simulink model "serial_communication_simulink_model"  (Simulink 7.9)
settings: Solver=ode45  StartTime=0.0  StopTime=10.0  RelTol=1e-3
undefined symbols (not defined in the file or in its folder): LF, serial
libraries: instrumentlib x2
settings Model: Creator=Alexandre  LastModifiedBy=Alexandre

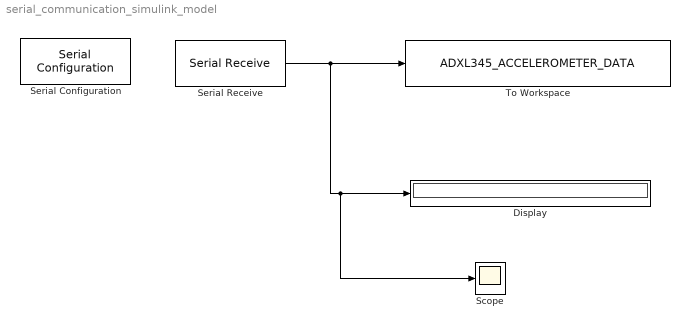
== system serial_communication_simulink_model ==
  Display : Display
  Scope : Scope
      settings: YMin=12.5  YMax=57.5
  Serial Configuration : instrumentlib/Serial Configuration  Priority=-200000  ComPortMenu=COM3  ComPort=COM3  ObjConstructor=serial('COM3');  BaudRate=9600  DataBits=8  Parity=none  StopBits=1  FlowControl=none  Timeout=10  ByteOrder=LittleEndian
  Serial Receive : instrumentlib/Serial Receive  ComPortMenu=COM3  ComPort=COM3  ObjConstructor=serial('COM3');  Terminator=LF ('\n')  DataSize="[1  3]"  DataType=uint8  EnableBlockingMode=on  ActionDataUnavailable=Output last received value  CustomValue=0  SampleTime=0.01
  To Workspace : ToWorkspace  VariableName=ADXL345_ACCELEROMETER_DATA  SampleTime=-1  SaveFormat=Structure With Time
  wires:
  Serial Receive/1 -> To Workspace/1, Display/1, Scope/1
